simulink model "ParallCellModel_ODE"  (R2025b)
settings: Solver=FixedStepAuto  StartTime=0.0  StopTime=5400  FixedStep=1  RelTol=1e-3
InitFcn:
  | InitParameterParallModel
undefined symbols (not defined in the file or in its folder): par_model
libraries: matrix_library x3
settings Model: Creator=Steven  LastModifiedBy=franzwendel
settings SolverCC: AlgebraicLoopSolver=TrustRegion
settings DataIOCC: ReturnWorkspaceOutputs=off
settings DebuggingCC: UnconnectedInputMsg=warning  UnconnectedOutputMsg=warning  UnconnectedLineMsg=warning  ArithmeticOperatorsInVariantConditions=warning
settings ModelReferenceCC: EnableRefExpFcnMdlSchedulingChecks=on
settings SFSimCC: SimUseLocalCustomCode=off  CustomCodeUndefinedFunction=UseInterfaceOnly
settings RTWCC: RTWUseLocalCustomCode=off  GPUComputeCapability=3.5  DLArmComputeVersion=19.05
settings ConfigComp: DVMaxProcessTime=300.0  DVMaxTestCaseSteps=10000.0  DVTestSuiteOptimization=Auto  DVAbsoluteTolerance=1.0e-5  DVDefectChecker=off  DVDetectOutOfBounds=on  DVMaxViolationSteps=20.0  DVHarnessSource=Signal Editor  DVActiveTab=0.0

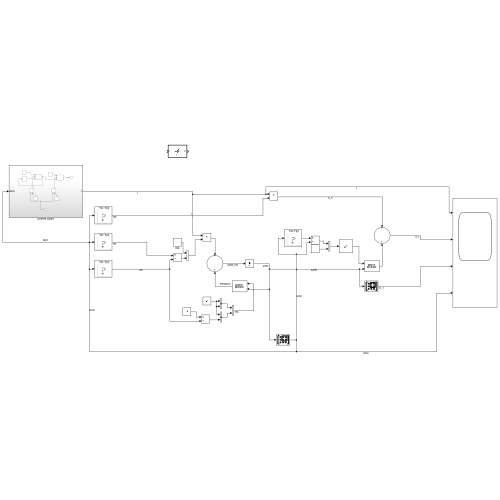
[thumbnail: Simulink's stored preview of the top-level diagram]
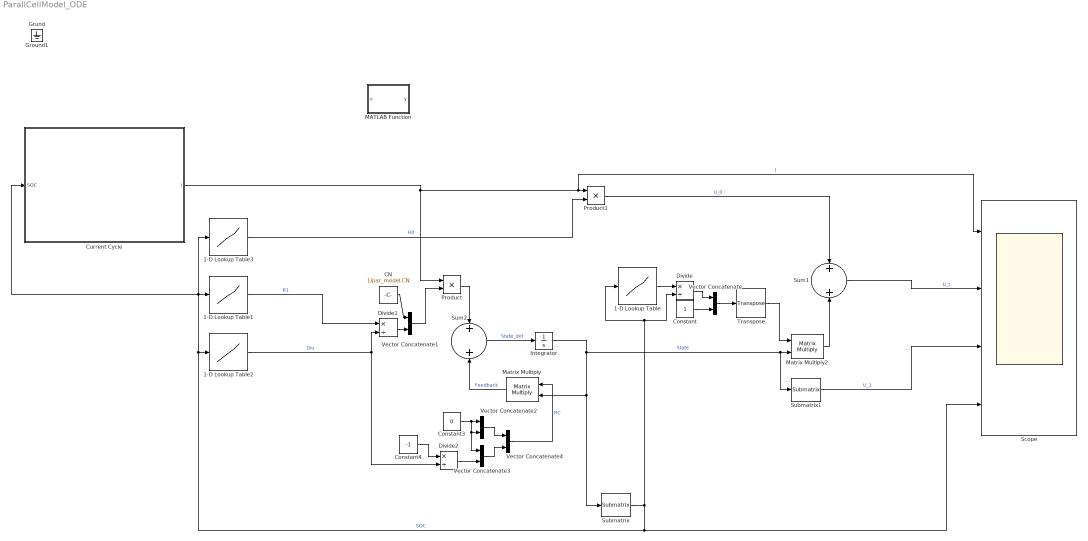
== system ParallCellModel_ODE ==
  1-D Lookup Table : Lookup_n-D  NumberOfTableDimensions=1  BreakpointsForDimension1=par_model.Data.SOC  Table=par_model.Data.OCV  InternalRulePriority=Speed  RndMeth=Simplest
  1-D Lookup Table1 : Lookup_n-D  NumberOfTableDimensions=1  BreakpointsForDimension1=par_model.SOC_Param  Table=par_model.R1  InternalRulePriority=Speed  RndMeth=Simplest
  1-D Lookup Table2 : Lookup_n-D  NumberOfTableDimensions=1  BreakpointsForDimension1=par_model.SOC_Param  Table=par_model.Tau1  InternalRulePriority=Speed  RndMeth=Simplest
  1-D Lookup Table3 : Lookup_n-D  NumberOfTableDimensions=1  BreakpointsForDimension1=par_model.SOC_Param  Table=par_model.R0  InternalRulePriority=Speed  RndMeth=Simplest
  CN : Constant  Value=1/par_model.CN
  Constant : Constant  VectorParams1D=off
  Constant3 : Constant  Value=0
  Constant4 : Constant  Value=-1
  Current Cycle : Subsystem
  Divide : Product  Inputs=*/
  Divide1 : Product  Inputs=*/
  Divide2 : Product  Inputs=*/
  Integrator : Integrator  InitialCondition=par_model.x_init
  MATLAB Function : MATLAB Function  TreatAsAtomicUnit=on
  Matrix Multiply : Product  Multiplication=Matrix(*)
  Matrix Multiply2 : Product  Multiplication=Matrix(*)
  Product : Product
  Product1 : Product
  Scope : Scope  NumInputPorts=4
      settings: ActiveDisplayYMinimum=-28.5390625  ActiveDisplayYMaximum=16.8515625
  Submatrix : matrix_library/Submatrix  RowSpan=One row  RowStartMode=First  RowStartIndex=1  RowEndMode=Last  RowEndIndex=1  ColSpan=One column  ColStartMode=First  ColStartIndex=1  ColEndMode=Last  ColEndIndex=1
  Submatrix1 : matrix_library/Submatrix  RowSpan=One row  RowStartMode=Last  RowStartIndex=1  RowEndMode=Last  RowEndIndex=1  ColSpan=One column  ColStartMode=Last  ColStartIndex=1  ColEndMode=Last  ColEndIndex=1
  Sum1 : Sum
  Sum2 : Sum
  Transpose : matrix_library/Transpose
  Vector Concatenate : Concatenate  Mode=Multidimensional array
  Vector Concatenate1 : Concatenate  Mode=Multidimensional array
  Vector Concatenate2 : Concatenate
  Vector Concatenate3 : Concatenate
  Vector Concatenate4 : Concatenate  Mode=Multidimensional array  ConcatenateDimension=2
  Ground1 : Ground  IOType=siggen
  Grund : Ground  IOType=siggen
  wires:
  Sum1/1 -> Scope/2  "U_t"
  1-D Lookup Table/1 -> Divide/1
  Divide/1 -> Vector Concatenate/1
  Constant/1 -> Vector Concatenate/2
  CN/1 -> Vector Concatenate1/1
  1-D Lookup Table2/1 -> Divide2/2, Divide1/2  "tau"
  Divide1/1 -> Vector Concatenate1/2
  Constant3/1 -> Vector Concatenate3/1, Vector Concatenate2/2, Vector Concatenate2/1
  Vector Concatenate2/1 -> Vector Concatenate4/1
  Vector Concatenate3/1 -> Vector Concatenate4/2
  Divide2/1 -> Vector Concatenate3/2
  Constant4/1 -> Divide2/1
  Vector Concatenate1/1 -> Product/2
  Submatrix/1 -> Divide/2, 1-D Lookup Table/1, 1-D Lookup Table3/1, Current Cycle/1(SOC), 1-D Lookup Table1/1, 1-D Lookup Table2/1, Scope/4  "SOC"
  1-D Lookup Table3/1 -> Product1/2  "R0"
  Vector Concatenate4/1 -> Matrix Multiply/1  "RC"
  Vector Concatenate/1 -> Transpose/1
  Transpose/1 -> Matrix Multiply2/1
  Matrix Multiply2/1 -> Sum1/2
  Sum2/1 -> Integrator/1  "State_dot"
  Integrator/1 -> Matrix Multiply2/2, Submatrix1/1, Submatrix/1, Matrix Multiply/2  "State"
  Product/1 -> Sum2/1
  Product1/1 -> Sum1/1  "U_0"
  Submatrix1/1 -> Scope/3  "U_1"
  Matrix Multiply/1 -> Sum2/2  "Feedback"
  1-D Lookup Table1/1 -> Divide1/1  "R1"
  Current Cycle/1(I) -> Scope/1, Product1/1, Product/1  "I"

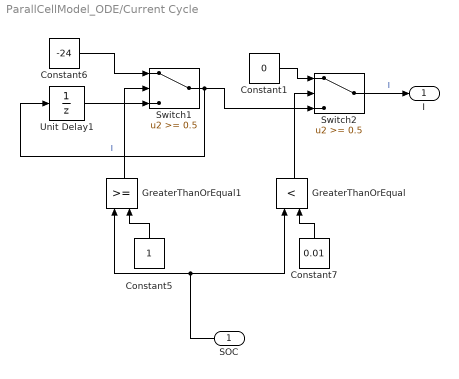
== system ParallCellModel_ODE/Current Cycle ==
  SOC : Inport
  Constant1 : Constant  Value=0  VectorParams1D=off
  Constant5 : Constant  VectorParams1D=off
  Constant6 : Constant  Value=-24  VectorParams1D=off
  Constant7 : Constant  Value=0.01  VectorParams1D=off
  GreaterThanOrEqual : RelationalOperator  Operator=<  OutDataTypeStr=boolean  RndMeth=Simplest  InputSameDT=off
  GreaterThanOrEqual1 : RelationalOperator  OutDataTypeStr=boolean  RndMeth=Simplest  InputSameDT=off
  Switch1 : Switch  Threshold=0.5  SaturateOnIntegerOverflow=off  InputSameDT=off
  Switch2 : Switch  Threshold=0.5  SaturateOnIntegerOverflow=off  InputSameDT=off
  Unit Delay1 : UnitDelay  InitialCondition=12.5 * par_model.eta_charge  SampleTime=-1  HasFrameUpgradeWarning=on
  I : Outport
  wires:
  Switch1/1 -> Switch2/3, Unit Delay1/1  "I"
  SOC/1 -> GreaterThanOrEqual/1, GreaterThanOrEqual1/1
  GreaterThanOrEqual1/1 -> Switch1/2
  Constant7/1 -> GreaterThanOrEqual/2
  Constant6/1 -> Switch1/1
  GreaterThanOrEqual/1 -> Switch2/2
  Constant5/1 -> GreaterThanOrEqual1/2
  Unit Delay1/1 -> Switch1/3
  Constant1/1 -> Switch2/1
  Switch2/1 -> I/1  "I"

== matlab function ParallCellModel_ODE/MATLAB Function ==
  data: u input; y output
function y = fcn(u)

y = u;
